simulink model "thermal_noise"  (R2025b)
settings: Solver=VariableStepAuto  StartTime=0.0  StopTime=10.0  RelTol=1e-3
settings Model: Creator=divya  LastModifiedBy=divya

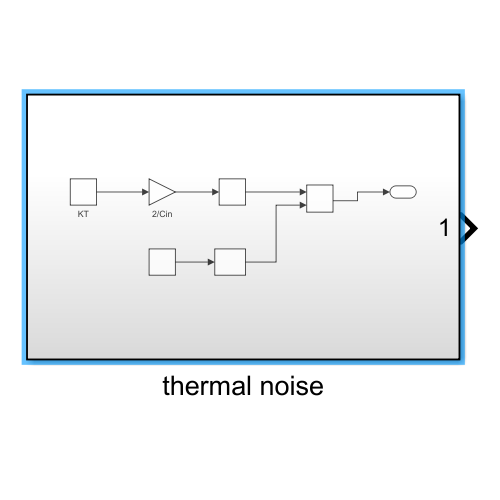
[thumbnail: Simulink's stored preview of the top-level diagram]
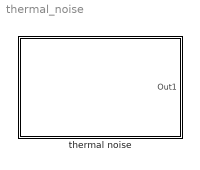
== system thermal_noise ==
  thermal noise : Subsystem

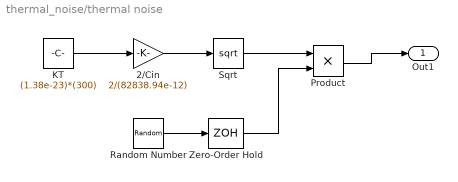
== system thermal_noise/thermal noise ==
  2/Cin : Gain  Gain=2/(82838.94e-12)
  KT : Constant  Value=(1.38e-23)*(300)
  Product : Product
  Random Number : RandomNumber  SampleTime=0.1
  Sqrt : Sqrt
  Zero-Order Hold : ZeroOrderHold  SampleTime=1/(2e3*128)
  Out1 : Outport
  wires:
  Product/1 -> Out1/1
  Random Number/1 -> Zero-Order Hold/1
  KT/1 -> 2/Cin/1
  Zero-Order Hold/1 -> Product/2
  2/Cin/1 -> Sqrt/1
  Sqrt/1 -> Product/1
